simulink subsystem "Create_LLA_from_States"  (R2023b)
settings: Solver=VariableStepAuto  StartTime=0.0  StopTime=10.0  RelTol=1e-3
undefined symbols (not defined in the file): Earth, m_to_mm, ref_height, WGS84
libraries: aerolibtransform2 x1
settings Model: Creator=The MathWorks, Inc.  LastModifiedBy=The MathWorks, Inc.
settings SolverCC: AlgebraicLoopSolver=TrustRegion
settings DebuggingCC: UnconnectedInputMsg=warning  UnconnectedOutputMsg=warning  UnconnectedLineMsg=warning
settings ModelReferenceCC: EnableRefExpFcnMdlSchedulingChecks=on
settings RTWCC: DLArmComputeVersion=19.05

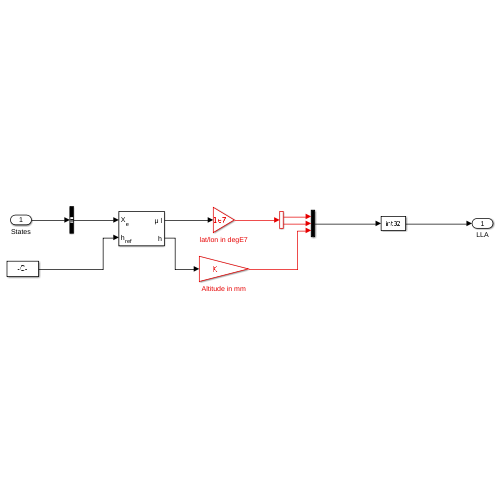
[thumbnail: Simulink's stored preview of the top-level diagram]
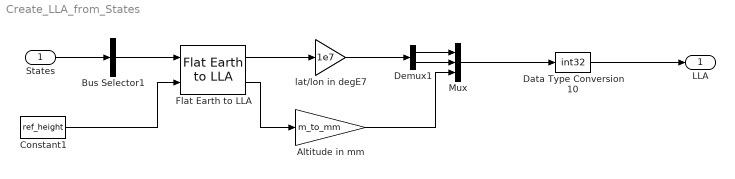
== system Create_LLA_from_States ==
  States : Inport
  Altitude in mm : Gain  Gain=m_to_mm
  Bus Selector1 : BusSelector  OutputSignals=X,Y,Z  OutputAsBus=on
  Constant1 : Constant  Value=ref_height  OutDataTypeStr=Inherit: Inherit via back propagation
  Data Type Conversion10 : DataTypeConversion  OutDataTypeStr=int32  SaturateOnIntegerOverflow=off  RndMeth=Floor
  Demux1 : Demux  Outputs=2
  Flat Earth to LLA : aerolibtransform2/Flat Earth to LLA  units=Metric (MKS)  ptype=Earth (WGS84)  F=1/298.257223563  R=6378137  refPosPort=off  LL0=[0 10]  psi=0
  Mux : Mux  Inputs=3
  lat/lon in degE7 : Gain  Gain=1e7
  LLA : Outport
  wires:
  lat/lon in degE7/1 -> Demux1/1
  Altitude in mm/1 -> Mux/3
  Mux/1 -> Data Type Conversion10/1
  Data Type Conversion10/1 -> LLA/1
  States/1 -> Bus Selector1/1
  Constant1/1 -> Flat Earth to LLA/2
  Demux1/2 -> Mux/2
  Flat Earth to LLA/2 -> Altitude in mm/1
  Flat Earth to LLA/1 -> lat/lon in degE7/1
  Demux1/1 -> Mux/1
  Bus Selector1/1 -> Flat Earth to LLA/1
